simulink model "sampleModel139"  (R2021b)
settings: Solver=VariableStepAuto  StartTime=0.0  StopTime=10.0  RelTol=1e-3
undefined symbols (not defined in the file or in its folder): DiscIntNeverNeededParam, Newton, Raphson
libraries: simulink x4, slpidlib x1
settings Model: Creator=user  LastModifiedBy=user

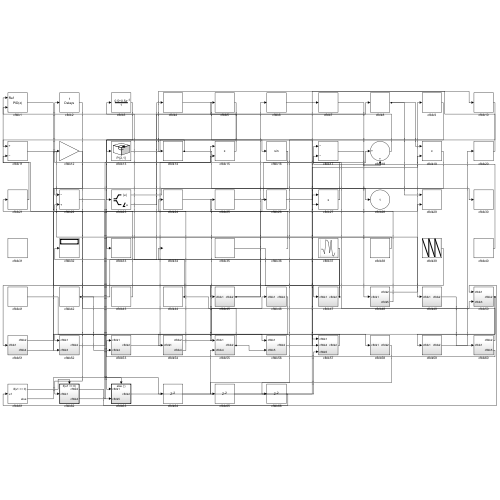
[thumbnail: Simulink's stored preview of the top-level diagram]
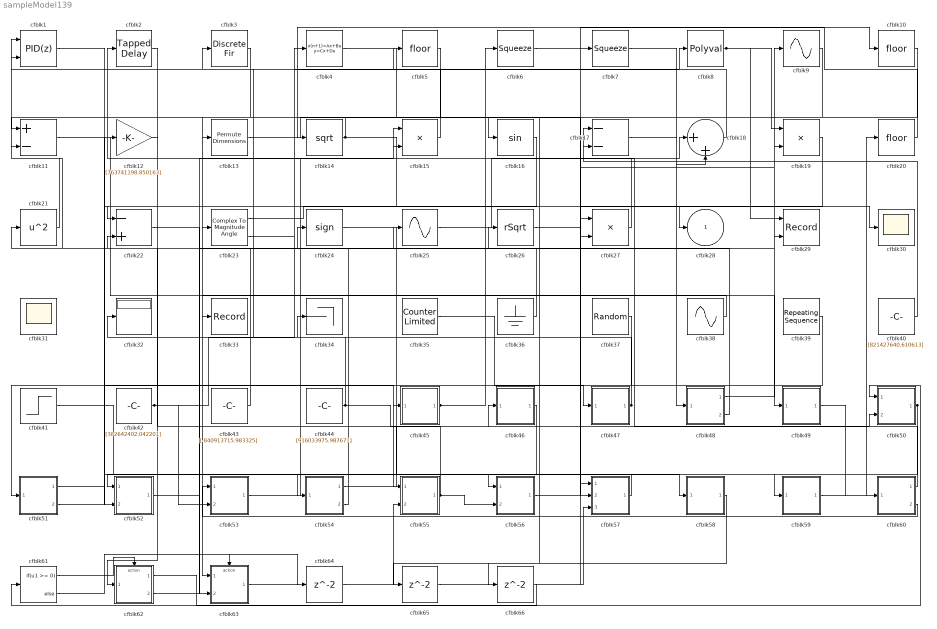
== system sampleModel139 ==
  cfblk1 : slpidlib/PID Controller (2DOF)  Controller=PID  Form=Parallel  TimeDomain=Discrete-time  UseExternalTs=off  SampleTime=1  IntegratorMethod=Forward Euler  FilterMethod=Forward Euler  ControllerParametersSource=internal  P=1  I=1  D=0  UseFilter=on  N=100  b=1  c=1  TunerSelectOption=Transfer Function Based (PID Tuner App)  InitialConditionSource=internal  InitialConditionForIntegrator=0  InitialConditionForFilter=0  DifferentiatorICPrevScaledInput=0  ExternalReset=none  TrackingMode=off  Kt=1  LimitOutput=off  SatLimitsSource=internal  UpperSaturationLimit=inf  LowerSaturationLimit=-inf  LinearizeAsGain=off  AntiWindupMode=none  Kb=1  POutMin=[]  POutMax=[]  IOutMin=[]  IOutMax=[]  DOutMin=[]  DOutMax=[]  NOutMin=[]  NOutMax=[]  bOutMin=[]  bOutMax=[]  cOutMin=[]  cOutMax=[]  SumOutMin=[]  SumOutMax=[]  SaturationOutMin=[]  SaturationOutMax=[]  PParamMin=[]  PParamMax=[]  IParamMin=[]  IParamMax=[]  DParamMin=[]  DParamMax=[]  NParamMin=[]  NParamMax=[]  bParamMin=[]  bParamMax=[]  cParamMin=[]  cParamMax=[]  KbParamMin=[]  KbParamMax=[]  KtParamMin=[]  KtParamMax=[]  KbOutMin=[]  KbOutMax=[]  KtOutMin=[]  KtOutMax=[]  IntegratorOutMin=[]  IntegratorOutMax=[]  FilterOutMin=[]  FilterOutMax=[]  SumI1OutMin=[]  SumI1OutMax=[]  SumI2OutMin=[]  SumI2OutMax=[]  SumI3OutMin=[]  SumI3OutMax=[]  SumI4OutMin=[]  SumI4OutMax=[]  SumDOutMin=[]  SumDOutMax=[]  Sum1OutMin=[]  Sum1OutMax=[]  Sum2OutMin=[]  Sum2OutMax=[]  Sum3OutMin=[]  Sum3OutMax=[]  DifferentiatorOutMin=[]  DifferentiatorOutMax=[]  FilterDiffOutCoefMin=[]  FilterDiffOutCoefMax=[]  ReciprocalOutMin=[]  ReciprocalOutMax=[]  SumDenOutMin=[]  SumDenOutMax=[]  SumNumOutMin=[]  SumNumOutMax=[]  DivideOutMin=[]  DivideOutMax=[]  UdiffTsProdOutMin=[]  UdiffTsProdOutMax=[]  NTsProdOutMin=[]  NTsProdOutMax=[]  UintegralTsProdOutMin=[]  UintegralTsProdOutMax=[]  UngainTsProdOutMin=[]  UngainTsProdOutMax=[]  IntegratorContinuousStateAttributes=''  IntegratorStateMustResolveToSignalObject=off  IntegratorRTWStateStorageClass=Auto  FilterContinuousStateAttributes=''  FilterStateMustResolveToSignalObject=off  FilterRTWStateStorageClass=Auto  ParallelPVariant=InternalParameters  IdealPVariant=Disabled  IVariant=InternalParameters  DVariant=InternalParameters  bVariant=InternalParameters  cVariant=InternalParameters  IntegratorVariant=Discrete  SatVariant=Disabled  AWVariant=Passthrough  PCopyVariant=Disabled  TRVariant=Disabled  FdbkBlocksVariant=Forward  IdealPFdbkVariant=Disabled  SatFdbkVariant=Disabled  DerivativeFilterVariant=ForwardEulerFilter  NVariant=InternalParameters  NCopyVariant=Disabled  FilterICVariant=InternalICsFilter  IntegratorICVariant=InternalICs  ExternalResetVariant=Disabled  TRSumVariant=Passthrough  SumFdbkVariant=Disabled  SumVariant=Sum_PID  TsampFilterVariant=InternalTs  TsampNgainVariant=Passthrough  TsampIntegralVariant=Passthrough  ExternalSaturationOutDataTypeStr=Inherit: Same as second input
      settings: SourceProductBaseCode=SL
  cfblk10 : Rounding
  cfblk11 : Sum  Inputs=+-
  cfblk12 : Gain  Gain=[763741198.850163]
  cfblk13 : PermuteDimensions
  cfblk14 : Sqrt  SaturateOnIntegerOverflow=on
  cfblk15 : Product  Inputs=**
  cfblk16 : Trigonometry
  cfblk17 : Sum  Inputs=--
  cfblk18 : Sum  Inputs=|++
  cfblk19 : Product  Inputs=**
  cfblk2 : simulink/Discrete/Tapped Delay  vinit=0.0  samptime=-1  NumDelays=1  DelayOrder=Oldest  includeCurrent=off
  cfblk20 : Rounding
  cfblk21 : Math  Operator=square  SaturateOnIntegerOverflow=on
  cfblk22 : Sum  Inputs=-+
  cfblk23 : ComplexToMagnitudeAngle
  cfblk24 : Signum
  cfblk25 : Sin  TimeSource=Use external signal  SampleTime=0
  cfblk26 : Sqrt  Operator=rSqrt  AlgorithmType=Newton-Raphson  SaturateOnIntegerOverflow=on
  cfblk27 : Product  Inputs=**
  cfblk29 : Record  FileSettingsInternal="{\"entries\":[{\"content\":{\"excelSettings\":{\"content\":{},\"type\":\"Streamout.ExcelSettings\"}},\"type\":\"Streamout.FileSettingStorage\",\"uuid\":\"035eb0ec-31ac-4015-9700-7ee30b468211\"}],\"packageUris\":[\"http://schema.mathworks.com/mf0/streamout_blocks/R2020a\"],\"version\":\"1.0\"}"  Layout=[1 1]  SignalsInternal="{\"entries\":[{\"content\":{\"signals\":[{\"content\":{\"blockPath\":[\"sampleModel139/cfblk29\"],\"channel\":[],\"dimensions\":[1],\"domain\":\"sampleModel139/cfblk29\",\"lineColor\":\"#a2142f\",\"plots\":[1],\"port\":1,\"sid\":[\"\"],\"signalID\":4965,\"signalName\":\"cfblk8\"},\"type\":\"RecordBlkView.Signal\",\"uuid\":\"c6bd2487-9314-43da-b1fb-71fc1f77a4db\"},{\"content\":{\"blockPath\":[\"sampleModel139/cfblk29\"],\"channel\":[],\"dimensions\":[1],\"domain\":\"sampleModel139/cfblk29\",\"lineColor\":\"#139fff\",\"plots\":[1],\"port\":2,\"sid\":[\"\"],\"signalID\":4969,\"signalName\":\"cfblk45\"},\"type\":\"RecordBlkView.Signal\",\"uuid\":\"26fe25fa-08c0-4ee0-9d54-8ed27315a8a5\"}]},\"type\":\"RecordBlkView.InputSignals\",\"uuid\":\"b772ec9c-d018-4776-880e-577078a360d2\"}],\"packageUris\":[\"http://schema.mathworks.com/mf0/streamout_blocks/R2020a\"],\"version\":\"1.0\"}"  VisualizationBindings="{\"xyplotplugin\":{\"info\":[{\"series\":[{\"bindingParametersList\":[{\"parameter\":\"X-Axis\",\"signalID\":4965,\"signalName\":\"cfblk8\"},{\"parameter\":\"Y-Axis\",\"signalID\":4969,\"signalName\":\"cfblk45\"}],\"seriesID\":37675}],\"subplotID\":1}]}}"  CompatibilityTag=XY
  cfblk3 : DiscreteFir  SampleTime=1
  cfblk30 : Scope
  cfblk31 : Scope
      settings: Floating=on
  cfblk32 : Display
  cfblk33 : Record  FileSettingsInternal="{\"entries\":[{\"content\":{\"excelSettings\":{\"content\":{},\"type\":\"Streamout.ExcelSettings\"}},\"type\":\"Streamout.FileSettingStorage\",\"uuid\":\"4e6fae24-c750-479a-bc5f-d2fa416f0b49\"}],\"packageUris\":[\"http://schema.mathworks.com/mf0/streamout_blocks/R2020a\"],\"version\":\"1.0\"}"  SignalsInternal="{\"entries\":[{\"content\":{\"signals\":[{\"content\":{\"blockPath\":[\"sampleModel139/cfblk33\"],\"channel\":[],\"dimensions\":[1],\"domain\":\"sampleModel139/cfblk33\",\"lineColor\":\"#64d413\",\"plots\":[1],\"port\":1,\"sid\":[\"\"],\"signalID\":4973,\"signalName\":\"cfblk38\"},\"type\":\"RecordBlkView.Signal\",\"uuid\":\"b933cee2-0ab4-4ff8-9a7b-ea3465a830b1\"}]},\"type\":\"RecordBlkView.InputSignals\",\"uuid\":\"fc2d5747-40b1-4522-9bd4-405ff4870c1d\"}],\"packageUris\":[\"http://schema.mathworks.com/mf0/streamout_blocks/R2020a\"],\"version\":\"1.0\"}"  VisualizationBindings="{\"sparklinesplugin\":{\"info\":[{\"bindingParametersList\":[],\"subplotID\":1}]}}"
  cfblk34 : Terminator
  cfblk35 : simulink/Sources/Counter Limited  uplimit=[105.000000]  tsamp=-1
  cfblk36 : Ground
  cfblk37 : RandomNumber  Mean=[-82458.859400]  Variance=[16732.506883]  Seed=[51619611.000000]  SampleTime=0.1
  cfblk38 : Sin  Amplitude=[758373332.756424]  Bias=[-342353249.313701]  SampleTime=0
  cfblk39 : simulink/Sources/Repeating Sequence  rep_seq_t=[0 2]  rep_seq_y=[313282713.751329, 100618207.473255]
  cfblk4 : DiscreteStateSpace
  cfblk40 : Constant  Value=[821427640.610613]  SampleTime=1
  cfblk41 : Step  Time=[22.000000]  Before=[502911261.959366]  After=[-124766894.085280]  SampleTime=0
  cfblk42 : Constant  Value=[382642402.042201]  SampleTime=1
  cfblk43 : Constant  Value=[-840913715.983325]  SampleTime=1
  cfblk44 : Constant  Value=[916033975.987671]  SampleTime=1
  cfblk45 : Subsystem
  cfblk46 : Subsystem
  cfblk47 : Subsystem
  cfblk48 : Subsystem
  cfblk49 : Subsystem
  cfblk5 : Rounding
  cfblk50 : Subsystem
  cfblk51 : Subsystem
  cfblk52 : Subsystem
  cfblk53 : Subsystem
  cfblk54 : Subsystem
  cfblk55 : Subsystem
  cfblk56 : Subsystem
  cfblk57 : Subsystem
  cfblk58 : Subsystem
  cfblk59 : Subsystem
  cfblk6 : Squeeze
  cfblk60 : Subsystem
  cfblk61 : If  IfExpression=u1 >= 0  SampleTime=1
  cfblk62 : Subsystem  TreatAsAtomicUnit=on
  cfblk63 : Subsystem  TreatAsAtomicUnit=on
  cfblk64 : Delay  SampleTime=1
  cfblk65 : Delay  SampleTime=1
  cfblk66 : Delay  SampleTime=1
  cfblk7 : Squeeze
  cfblk8 : Polyval  Coefs=[ +2.081618890e-019, -1.441693666e-014, +4.719686976e-010, -8.536869453e-006, +1.621573104e-001, -8.087801117e+001 ]
  cfblk9 : Sin  TimeSource=Use external signal  SampleTime=0
  cfblk28 : Outport
  wires:
  cfblk25/1 -> cfblk18/1
  cfblk13/1 -> cfblk16/1
  cfblk53/1(cfblk2) -> cfblk15/1
  cfblk49/1(cfblk2) -> cfblk60/1(cfblk1)
  cfblk24/1 -> cfblk58/1(cfblk1)
  cfblk40/1 -> cfblk17/1
  cfblk27/1 -> cfblk2/1
  cfblk59/1(cfblk2) -> cfblk20/1
  cfblk20/1 -> cfblk14/1
  cfblk4/1 -> cfblk57/1(cfblk1)
  cfblk45/1(cfblk2) -> cfblk6/1, cfblk29/2
  cfblk54/1(cfblk2) -> cfblk46/1(cfblk1)
  cfblk48/1(cfblk2) -> cfblk9/1
  cfblk56/1(cfblk2) -> cfblk7/1
  cfblk44/1 -> cfblk32/1, cfblk50/2(cfblk3)
  cfblk36/1 -> cfblk25/1
  cfblk17/1 -> cfblk48/1(cfblk1)
  cfblk11/1 -> cfblk49/1(cfblk1)
  cfblk50/1(cfblk2) -> cfblk57/2(cfblk4), cfblk59/1(cfblk1)
  cfblk21/1 -> cfblk1/1
  cfblk37/1 -> cfblk51/1(cfblk1)
  cfblk14/1 -> cfblk28/1, cfblk13/1
  cfblk47/1(cfblk2) -> cfblk34/1, cfblk3/1
  cfblk23/1 -> cfblk30/1
  cfblk39/1 -> cfblk55/1(cfblk1)
  cfblk7/1 -> cfblk18/2
  cfblk63/1(cfblk2) -> cfblk55/2(cfblk4)
  cfblk35/1 -> cfblk47/1(cfblk1)
  cfblk3/1 -> cfblk63/1(cfblk1)
  cfblk5/1 -> cfblk11/1
  cfblk42/1 -> cfblk4/1, cfblk53/2(cfblk4)
  cfblk18/1 -> cfblk5/1
  cfblk19/1 -> cfblk27/2
  cfblk38/1 -> cfblk33/1
  cfblk46/1(cfblk2) -> cfblk52/1(cfblk1)
  cfblk62/1(cfblk2) -> cfblk50/1(cfblk1)
  cfblk60/1(cfblk2) -> cfblk17/2
  cfblk60/2(cfblk5) -> cfblk53/1(cfblk1)
  cfblk51/1(cfblk2) -> cfblk12/1
  cfblk2/1 -> cfblk22/1
  cfblk57/1(cfblk2) -> cfblk54/1(cfblk1)
  cfblk54/2(cfblk4) -> cfblk24/1
  cfblk62/2(cfblk4) -> cfblk15/2
  cfblk8/1 -> cfblk19/1, cfblk29/1
  cfblk6/1 -> cfblk10/1
  cfblk12/1 -> cfblk62/1(cfblk1)
  cfblk48/2(cfblk5) -> cfblk21/1
  cfblk26/1 -> cfblk19/2
  cfblk15/1 -> cfblk1/2
  cfblk16/1 -> cfblk52/2(cfblk3)
  cfblk51/2(cfblk4) -> cfblk56/1(cfblk1)
  cfblk41/1 -> cfblk63/2(cfblk5)
  cfblk10/1 -> cfblk23/1
  cfblk43/1 -> cfblk11/2
  cfblk55/1(cfblk2) -> cfblk22/2, cfblk56/2(cfblk5)
  cfblk52/1(cfblk2) -> cfblk26/1
  cfblk1/1 -> cfblk45/1(cfblk1)
  cfblk23/2 -> cfblk8/1
  cfblk61/1 -> cfblk62/Action
  cfblk61/2 -> cfblk63/Action
  cfblk22/1 -> cfblk64/1
  cfblk64/1 -> cfblk27/1
  cfblk58/1(cfblk2) -> cfblk65/1
  cfblk65/1 -> cfblk57/3(cfblk5)
  cfblk9/1 -> cfblk66/1
  cfblk66/1 -> cfblk61/1

== system sampleModel139/cfblk45 ==
  cfblk1 : Inport
  cfblk3 : Bias  Bias=[-543554504.013159]
  cfblk2 : Outport
  wires:
  cfblk1/1 -> cfblk3/1
  cfblk3/1 -> cfblk2/1

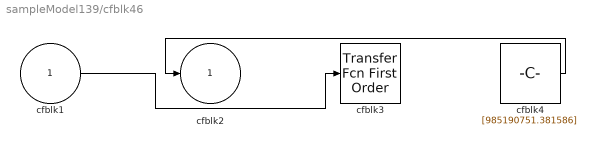
== system sampleModel139/cfblk46 ==
  cfblk1 : Inport
  cfblk3 : simulink/Discrete/Transfer Fcn First Order  PoleZ=0.95  ICPrevOutput=0.0  DoSatur=off
  cfblk4 : Constant  Value=[985190751.381586]  SampleTime=1
  cfblk2 : Outport
  wires:
  cfblk4/1 -> cfblk2/1
  cfblk1/1 -> cfblk3/1

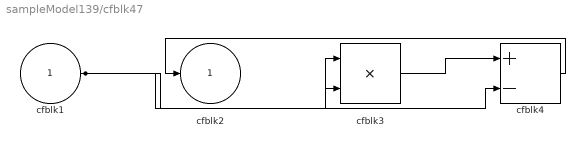
== system sampleModel139/cfblk47 ==
  cfblk1 : Inport
  cfblk3 : Product
  cfblk4 : Sum  Inputs=+-
  cfblk2 : Outport
  wires:
  cfblk3/1 -> cfblk4/1
  cfblk4/1 -> cfblk2/1
  cfblk1/1 -> cfblk3/1, cfblk4/2, cfblk3/2

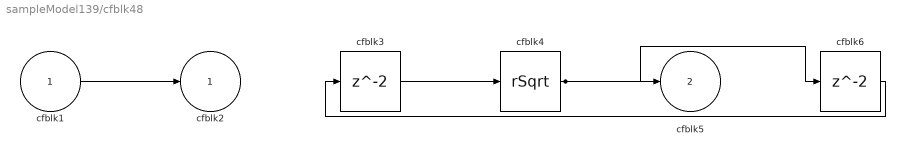
== system sampleModel139/cfblk48 ==
  cfblk1 : Inport
  cfblk3 : Delay  SampleTime=1
  cfblk4 : Sqrt  Operator=rSqrt  AlgorithmType=Newton-Raphson  SaturateOnIntegerOverflow=on
  cfblk6 : Delay  SampleTime=1
  cfblk2 : Outport
  cfblk5 : Outport  Port=2
  wires:
  cfblk1/1 -> cfblk2/1
  cfblk4/1 -> cfblk5/1, cfblk6/1
  cfblk3/1 -> cfblk4/1
  cfblk6/1 -> cfblk3/1

== system sampleModel139/cfblk49 ==
  cfblk1 : Inport
  cfblk3 : DiscreteFir  SampleTime=1
  cfblk2 : Outport
  wires:
  cfblk1/1 -> cfblk3/1
  cfblk3/1 -> cfblk2/1

== system sampleModel139/cfblk50 ==
  cfblk1 : Inport
  cfblk3 : Inport  Port=2
  cfblk2 : Outport
  wires:
  cfblk3/1 -> cfblk2/1

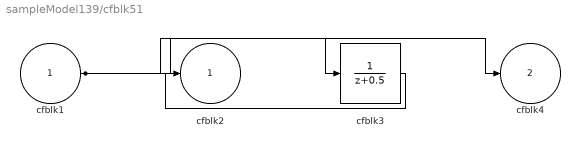
== system sampleModel139/cfblk51 ==
  cfblk1 : Inport
  cfblk3 : DiscreteTransferFcn  SampleTime=1
  cfblk2 : Outport
  cfblk4 : Outport  Port=2
  wires:
  cfblk1/1 -> cfblk3/1, cfblk4/1
  cfblk3/1 -> cfblk2/1

== system sampleModel139/cfblk52 ==
  cfblk1 : Inport
  cfblk3 : Inport  Port=2
  cfblk2 : Outport
  wires:
  cfblk3/1 -> cfblk2/1

== system sampleModel139/cfblk53 ==
  cfblk1 : Inport
  cfblk4 : Inport  Port=2
  cfblk3 : Assignment  DiagnosticForDimensions=Warning  IndexOptions=Index vector (dialog)  Indices=1  OutputSizes=1
  cfblk2 : Outport
  wires:
  cfblk4/1 -> cfblk2/1
  cfblk1/1 -> cfblk3/1, cfblk3/2

== system sampleModel139/cfblk54 ==
  cfblk1 : Inport
  cfblk3 : Product
  cfblk2 : Outport
  cfblk4 : Outport  Port=2
  wires:
  cfblk3/1 -> cfblk4/1
  cfblk1/1 -> cfblk2/1, cfblk3/1, cfblk3/2

== system sampleModel139/cfblk55 ==
  cfblk1 : Inport
  cfblk4 : Inport  Port=2
  cfblk3 : Constant  Value=[-65098958.715037]  SampleTime=1
  cfblk2 : Outport
  wires:
  cfblk1/1 -> cfblk2/1

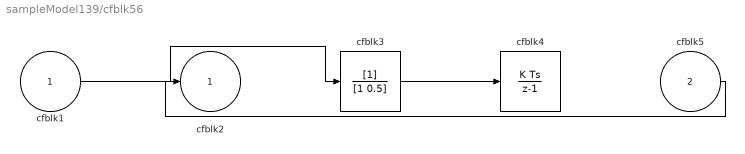
== system sampleModel139/cfblk56 ==
  cfblk1 : Inport
  cfblk5 : Inport  Port=2
  cfblk3 : DiscreteFilter  SampleTime=1
  cfblk4 : DiscreteIntegrator  ICPrevOutput=DiscIntNeverNeededParam  ICPrevScaledInput=DiscIntNeverNeededParam
  cfblk2 : Outport
  wires:
  cfblk3/1 -> cfblk4/1
  cfblk1/1 -> cfblk3/1
  cfblk5/1 -> cfblk2/1

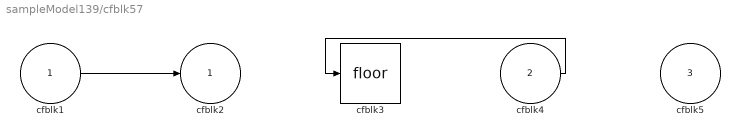
== system sampleModel139/cfblk57 ==
  cfblk1 : Inport
  cfblk4 : Inport  Port=2
  cfblk5 : Inport  Port=3
  cfblk3 : Rounding
  cfblk2 : Outport
  wires:
  cfblk1/1 -> cfblk2/1
  cfblk4/1 -> cfblk3/1

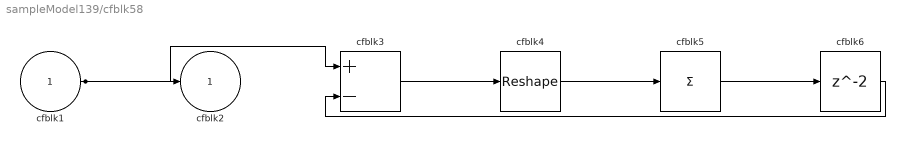
== system sampleModel139/cfblk58 ==
  cfblk1 : Inport
  cfblk3 : Sum  Inputs=+-
  cfblk4 : Reshape
  cfblk5 : Sum  Inputs=+
  cfblk6 : Delay  SampleTime=1
  cfblk2 : Outport
  wires:
  cfblk3/1 -> cfblk4/1
  cfblk1/1 -> cfblk3/1, cfblk2/1
  cfblk4/1 -> cfblk5/1
  cfblk5/1 -> cfblk6/1
  cfblk6/1 -> cfblk3/2

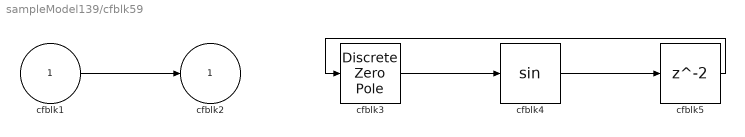
== system sampleModel139/cfblk59 ==
  cfblk1 : Inport
  cfblk3 : DiscreteZeroPole  Poles=[0 0.5]  Gain=1
  cfblk4 : Trigonometry
  cfblk5 : Delay  SampleTime=1
  cfblk2 : Outport
  wires:
  cfblk3/1 -> cfblk4/1
  cfblk1/1 -> cfblk2/1
  cfblk4/1 -> cfblk5/1
  cfblk5/1 -> cfblk3/1

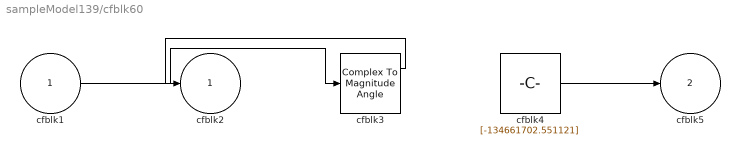
== system sampleModel139/cfblk60 ==
  cfblk1 : Inport
  cfblk3 : ComplexToMagnitudeAngle
  cfblk4 : Constant  Value=[-134661702.551121]  SampleTime=1
  cfblk2 : Outport
  cfblk5 : Outport  Port=2
  wires:
  cfblk4/1 -> cfblk5/1
  cfblk1/1 -> cfblk3/1
  cfblk3/1 -> cfblk2/1

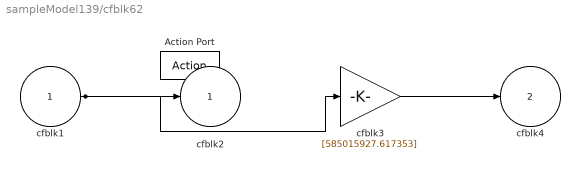
== system sampleModel139/cfblk62 ==
  cfblk1 : Inport
  Action Port : ActionPort  ActionPortLabel=if(u1 >= 0)
  cfblk3 : Gain  Gain=[585015927.617353]
  cfblk2 : Outport
  cfblk4 : Outport  Port=2
  wires:
  cfblk1/1 -> cfblk2/1, cfblk3/1
  cfblk3/1 -> cfblk4/1

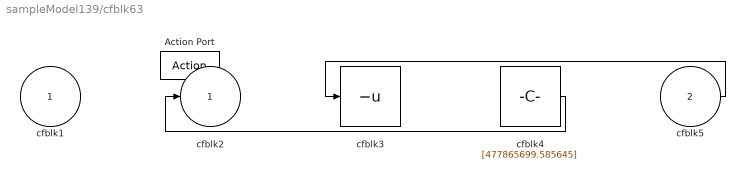
== system sampleModel139/cfblk63 ==
  cfblk1 : Inport
  cfblk5 : Inport  Port=2
  Action Port : ActionPort  ActionPortLabel=else
  cfblk3 : UnaryMinus
  cfblk4 : Constant  Value=[477865699.585645]  SampleTime=1
  cfblk2 : Outport
  wires:
  cfblk4/1 -> cfblk2/1
  cfblk5/1 -> cfblk3/1
